simulink model "quartersusp"  (R2019a)
settings: Solver=VariableStepAuto  StartTime=0.0  StopTime=50  RelTol=1e-4
values from neighbouring files (symbols this model uses):
  b1 = 350    [quartersusp_tf.m]
  b2 = 15020    [quartersusp_tf.m]
  k1 = 80000    [quartersusp_tf.m]
  k2 = 500000    [quartersusp_tf.m]
  m1 = 2500    [quartersusp_tf.m]
  m2 = 320    [quartersusp_tf.m]
settings Model: Creator=dağlar  LastModifiedBy=dağlar
settings DataIOCC: ReturnWorkspaceOutputs=off

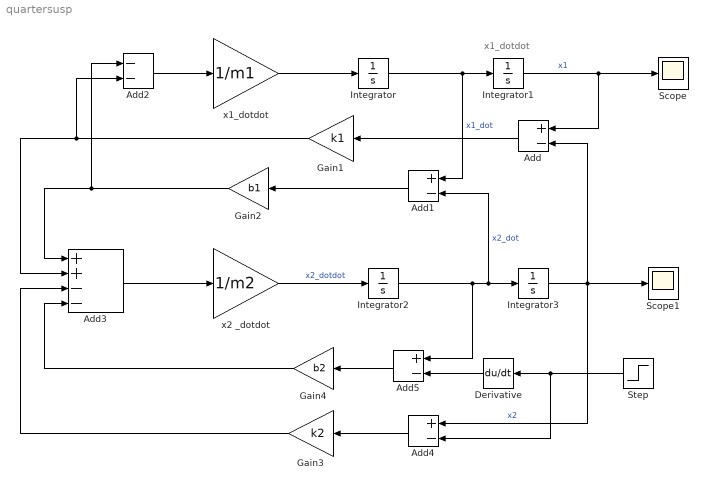
== system quartersusp ==
  note: x1_dotdot
  Add{,1,4..5} (4 alike) : Sum  Inputs=+-
  Add2 : Sum  Inputs=--
  Add3 : Sum  Inputs=++--
  Derivative : Derivative
  Gain1 : Gain  Gain=k1
  Gain2 : Gain  Gain=b1
  Gain3 : Gain  Gain=k2
  Gain4 : Gain  Gain=b2
  Integrator{,1..3} (4 alike) : Integrator
  Scope : Scope
  Scope1 : Scope
  Step : Step  Time=0  SampleTime=0
  x1_dotdot : Gain  Gain=1/m1
  "x2 _dotdot " : Gain  Gain=1/m2
  wires:
  Add3/1 -> "x2 _dotdot "/1
  Derivative/1 -> Add5/2
  Add2/1 -> x1_dotdot/1
  Gain2/1 -> Add2/1, Add3/1
  Integrator1/1 -> Add/1, Scope/1  "x1"
  Add/1 -> Gain1/1
  x1_dotdot/1 -> Integrator/1
  Integrator3/1 -> Scope1/1, Add/2, Add4/1  "x2"
  Gain3/1 -> Add3/3
  "x2 _dotdot "/1 -> Integrator2/1  "x2_dotdot"
  Gain4/1 -> Add3/4
  Add5/1 -> Gain4/1
  Add1/1 -> Gain2/1
  Add4/1 -> Gain3/1
  Integrator/1 -> Add1/1, Integrator1/1  "x1_dot"
  Integrator2/1 -> Add5/1, Integrator3/1, Add1/2  "x2_dot"
  Gain1/1 -> Add2/2, Add3/2
  Step/1 -> Add4/2, Derivative/1
